simulink model "HopperPlant_Old"  (R2023b)
settings: Solver=VariableStepAuto  StartTime=0.0  StopTime=100  RelTol=1e-3
libraries: slpidlib x5, aerolibsim3d x2, shared6dof x1, sim3dlib x1
settings Model: Creator=xavie  LastModifiedBy=xavie

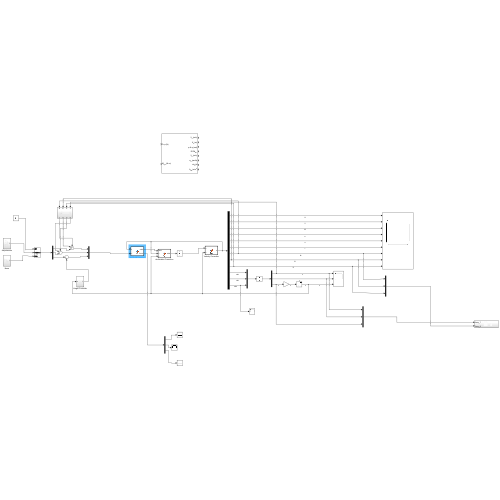
[thumbnail: Simulink's stored preview of the top-level diagram]
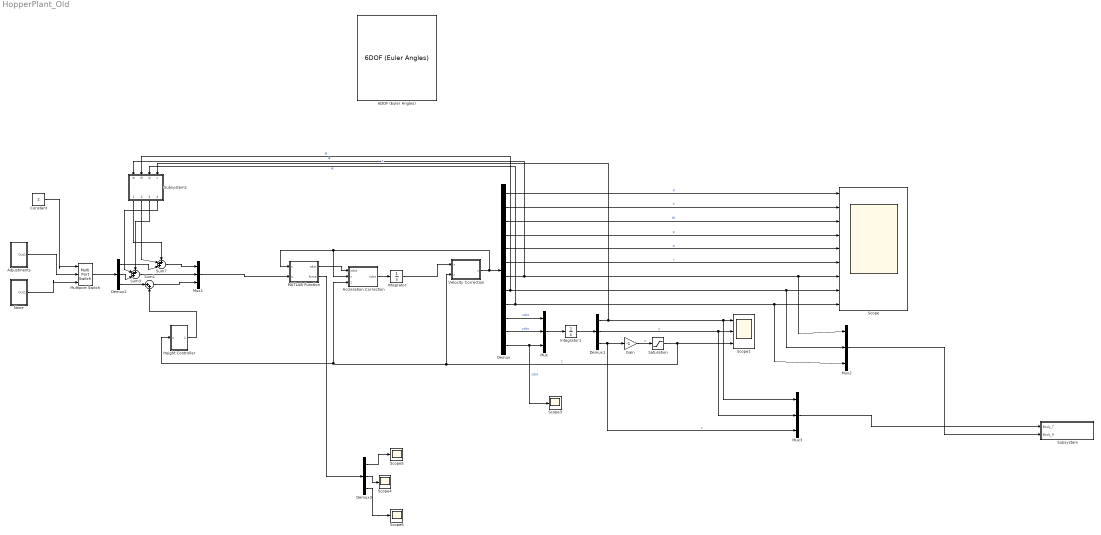
== system HopperPlant_Old ==
  6DOF (Euler Angles) : shared6dof/6DOF (Euler Angles)  units=Metric (MKS)  mtype=Fixed  rep=Euler Angles  xme_0=[0 0 0]  Vm_0=[0 0 0]  eul_0=[0 0 0]  pm_0=[0 0 0]  mass_0=1.0  mass_e=0.5  mass_f=2.0  inertia=eye(3)  inertia_e=eye(3)  inertia_f=2*eye(3)  k_quat=1.0  vre_flag=on  abi_flag=off  aMode=0  xme_statename=''  Vm_statename=''  eul_statename=''  quat_statename=''  pm_statename=''  mass_statename=''
  Accleration Correction : MATLAB Function  TreatAsAtomicUnit=on
  Adjustments : Subsystem
  Constant : Constant  Value=2
  Demux : Demux  Outputs=12
  Demux1 : Demux  Outputs=3
  Demux2 : Demux  Outputs=3
  Demux3 : Demux  Outputs=3
  Gain : Gain  Gain=-1
  Height Controller : Subsystem
  Integrator : Integrator  InitialCondition=[0;0;0;0;0;0;0;0;0;0;0;0]
  Integrator1 : Integrator  InitialCondition=[0;0;0]
  MATLAB Function : MATLAB Function  TreatAsAtomicUnit=on
  Multiport Switch : MultiPortSwitch  Inputs=2  SaturateOnIntegerOverflow=off  InputSameDT=off
  Mux{,1..3} (4 alike) : Mux  Inputs=3
  None : Subsystem
  Saturation : Saturate  UpperLimit=10000000000000000000000000000000000000000000  LowerLimit=0
  Scope : Scope  NumInputPorts=9
  Scope1 : Scope  NumInputPorts=3
  Scope{3..6} (4 alike) : Scope
  Subsystem : Subsystem
  Subsystem1 : Subsystem
  Sum1 : Sum  Inputs=|++
  Sum3 : Sum  Inputs=+++|
  Sum7 : Sum  Inputs=+++|
  Velocity Correction : MATLAB Function  TreatAsAtomicUnit=on
  wires:
  MATLAB Function/1(xdot) -> Accleration Correction/1("xdot ")
  Integrator/1 -> Velocity Correction/1("x ")
  Demux/1 -> Scope/1  "U"
  Demux/2 -> Scope/2  "V"
  Demux/3 -> Scope/3  "W"
  Demux/4 -> Scope/4  "p"
  Demux/5 -> Scope/5  "q"
  Demux/6 -> Scope/6  "r"
  Demux/7 -> Mux2/1, Scope/7, Subsystem1/1(Φ)  "Φ"
  Demux/8 -> Mux2/2, Scope/8, Subsystem1/2(Θ)  "Θ"
  Demux/9 -> Mux2/3, Scope/9, Subsystem1/3(Ψ)  "Ψ"
  Demux/10 -> Mux/1  "xdot"
  Demux/11 -> Mux/2  "ydot"
  Demux/12 -> Scope3/1, Mux/3  "zdot"
  Mux/1 -> Integrator1/1
  Integrator1/1 -> Demux1/1
  Demux1/1 -> Mux3/1, Scope1/1, Subsystem1/4(x)  "x"
  Demux1/2 -> Mux3/2, Scope1/2  "y"
  Demux1/3 -> Mux3/3, Gain/1  "z"
  Gain/1 -> Saturation/1  "z"
  Accleration Correction/1(xdot) -> Integrator/1
  Saturation/1 -> Velocity Correction/2(z), Height Controller/1(z), Accleration Correction/3(z), Scope1/3  "z"
  Velocity Correction/1(x) -> Accleration Correction/2(x), MATLAB Function/1(x), Demux/1
  Constant/1 -> Multiport Switch/1
  Adjustments/1(Out1) -> Multiport Switch/2
  None/1(Out1) -> Multiport Switch/3
  Multiport Switch/1 -> Demux2/1
  Demux2/3 -> Sum1/1
  Mux1/1 -> MATLAB Function/2(u)
  Sum1/1 -> Mux1/3
  MATLAB Function/2(force) -> Demux3/1
  Demux3/2 -> Scope4/1
  Demux3/1 -> Scope5/1
  Demux3/3 -> Scope6/1
  Mux2/1 -> Subsystem/2(Body_R)
  Mux3/1 -> Subsystem/1(Body_T)
  Sum3/1 -> Mux1/2
  Demux2/2 -> Sum3/3
  Demux2/1 -> Sum7/3
  Sum7/1 -> Mux1/1
  Height Controller/1(Out1) -> Sum1/2
  Subsystem1/1(Out1) -> Sum7/1
  Subsystem1/2(Out2) -> Sum7/2
  Subsystem1/3(Out3) -> Sum3/1
  Subsystem1/4(Out4) -> Sum3/2

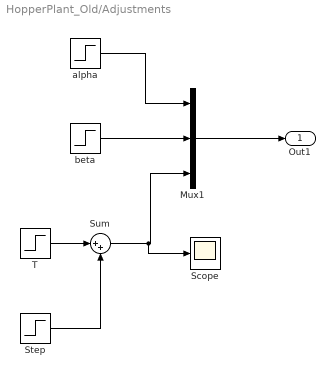
== system HopperPlant_Old/Adjustments ==
  Mux1 : Mux  Inputs=3
  Scope : Scope
  Step : Step  Time=10  After=-1500  SampleTime=0
  Sum : Sum  Inputs=|++
  T : Step  Time=0  After=1500  SampleTime=0
  alpha : Step  Time=0  After=pi/2  SampleTime=0
  beta : Step  Time=0  After=pi/2.001  SampleTime=0
  Out1 : Outport
  wires:
  alpha/1 -> Mux1/1
  Mux1/1 -> Out1/1
  beta/1 -> Mux1/2
  T/1 -> Sum/1
  Step/1 -> Sum/2
  Sum/1 -> Scope/1, Mux1/3

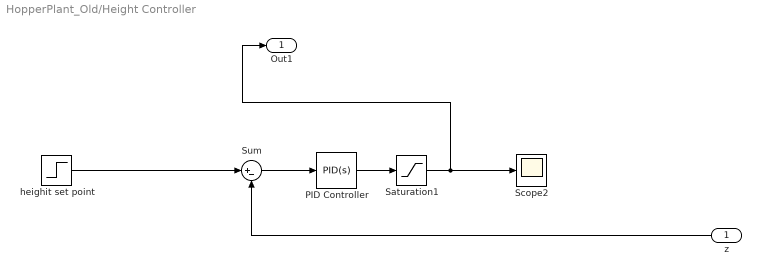
== system HopperPlant_Old/Height Controller ==
  z : Inport
  PID Controller : slpidlib/PID Controller  Controller=PID  Form=Parallel  TimeDomain=Continuous-time  UseExternalTs=off  SampleTime=-1  IntegratorMethod=Forward Euler  FilterMethod=Forward Euler  ControllerParametersSource=internal  P=40  I=2.1  UseKiTs=off  D=73  N=100  UseFilter=on  TunerSelectOption=Transfer Function Based (PID Tuner App)  InitialConditionSource=internal  InitialConditionForIntegrator=0  InitialConditionForFilter=0  DifferentiatorICPrevScaledInput=0  ExternalReset=none  TrackingMode=off  Kt=1  LimitOutput=off  SatLimitsSource=internal  UpperSaturationLimit=inf  LowerSaturationLimit=-inf  LinearizeAsGain=on  AntiWindupMode=none  Kb=1  LimitIntegrator=off  UpperIntegratorSaturationLimit=inf  LowerIntegratorSaturationLimit=-inf  POutMin=[]  POutMax=[]  IOutMin=[]  IOutMax=[]  DOutMin=[]  DOutMax=[]  NOutMin=[]  NOutMax=[]  SumOutMin=[]  SumOutMax=[]  SaturationOutMin=[]  SaturationOutMax=[]  PParamMin=[]  PParamMax=[]  IParamMin=[]  IParamMax=[]  DParamMin=[]  DParamMax=[]  NParamMin=[]  NParamMax=[]  KbParamMin=[]  KbParamMax=[]  KtParamMin=[]  KtParamMax=[]  KbOutMin=[]  KbOutMax=[]  KtOutMin=[]  KtOutMax=[]  IntegratorOutMin=[]  IntegratorOutMax=[]  FilterOutMin=[]  FilterOutMax=[]  SumI1OutMin=[]  SumI1OutMax=[]  SumI2OutMin=[]  SumI2OutMax=[]  SumI3OutMin=[]  SumI3OutMax=[]  SumI4OutMin=[]  SumI4OutMax=[]  SumDOutMin=[]  SumDOutMax=[]  DifferentiatorOutMin=[]  DifferentiatorOutMax=[]  FilterDiffOutCoefMin=[]  FilterDiffOutCoefMax=[]  ReciprocalOutMin=[]  ReciprocalOutMax=[]  SumDenOutMin=[]  SumDenOutMax=[]  SumNumOutMin=[]  SumNumOutMax=[]  DivideOutMin=[]  DivideOutMax=[]  UdiffTsProdOutMin=[]  UdiffTsProdOutMax=[]  NTsProdOutMin=[]  NTsProdOutMax=[]  UintegralTsProdOutMin=[]  UintegralTsProdOutMax=[]  UngainTsProdOutMin=[]  UngainTsProdOutMax=[]  ClampingZeroOutDataTypeStr=Inherit: Inherit via back propagation  ClampingZeroOutMin=[]  ClampingZeroOutMax=[]  FilterDenConstantOutDataTypeStr=Inherit: Inherit via back propagation  FilterDenConstantOutMin=[]  FilterDenConstantOutMax=[]  PCopyOutDataTypeStr=Inherit: Inherit via back propagation  PCopyOutMin=[]  PCopyOutMax=[]  NCopyOutDataTypeStr=Inherit: Inherit via back propagation  NCopyOutMin=[]  NCopyOutMax=[]  IntegratorContinuousStateAttributes=''  IntegratorStateMustResolveToSignalObject=off  IntegratorRTWStateStorageClass=Auto  FilterContinuousStateAttributes=''  FilterStateMustResolveToSignalObject=off  FilterRTWStateStorageClass=Auto  ParallelPVariant=InternalParameters  IdealPVariant=Disabled  IVariant=InternalParameters  DVariant=InternalParameters  IntegratorVariant=Continuous  SatVariant=Disabled  AWVariant=Passthrough  PCopyVariant=Disabled  TRVariant=Disabled  FdbkBlocksVariant=Forward  IdealPFdbkVariant=Disabled  SatFdbkVariant=Disabled  DerivativeFilterVariant=ContFilter  NVariant=InternalParameters  NCopyVariant=Disabled  FilterICVariant=InternalICsFilter  IntegratorICVariant=InternalICs  ExternalResetVariant=Disabled  TRSumVariant=Passthrough  SumFdbkVariant=Disabled  SumVariant=Sum_PID  TsampFilterVariant=InternalTs  TsampNgainVariant=Passthrough  TsampIntegralVariant=Disabled_SignalSpec  ExternalSaturationOutDataTypeStr=Inherit: Same as second input
  Saturation1 : Saturate  UpperLimit=1500  LowerLimit=0
  Scope2 : Scope
  Sum : Sum  Inputs=|+-
  heighit set point : Step  After=100  SampleTime=0
  Out1 : Outport
  wires:
  Saturation1/1 -> Out1/1, Scope2/1
  PID Controller/1 -> Saturation1/1
  Sum/1 -> PID Controller/1
  heighit set point/1 -> Sum/1
  z/1 -> Sum/2

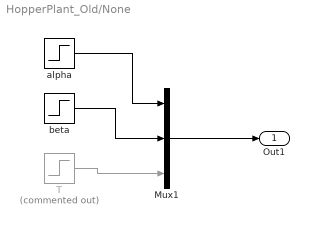
== system HopperPlant_Old/None ==
  Mux1 : Mux  Inputs=3
  T : Step  Commented=on  After=0  SampleTime=0
  alpha : Step  Time=0  After=0  SampleTime=0
  beta : Step  Time=0  After=pi/2.001  SampleTime=0
  Out1 : Outport
  wires:
  beta/1 -> Mux1/2
  T/1 -> Mux1/3
  alpha/1 -> Mux1/1
  Mux1/1 -> Out1/1

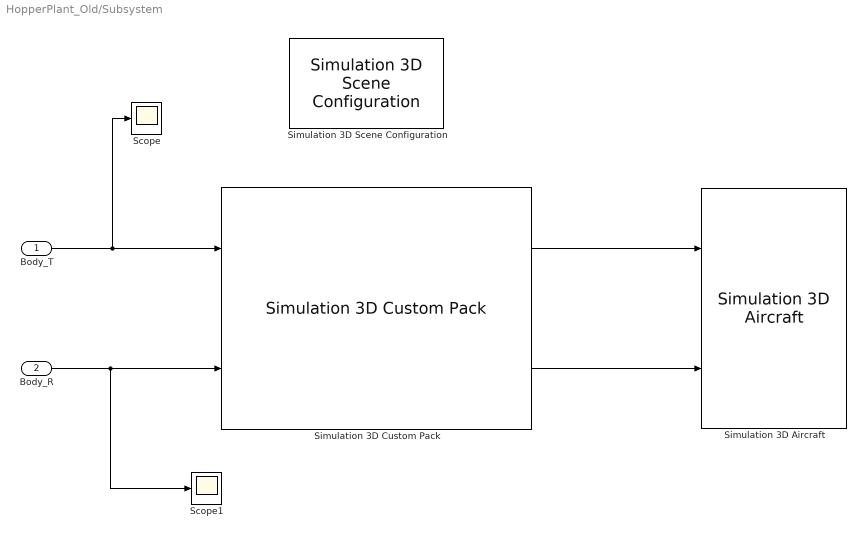
== system HopperPlant_Old/Subsystem ==
  Body_T : Inport
  Body_R : Inport  Port=2
  Scope : Scope
  Scope1 : Scope
  Simulation 3D Aircraft : aerolibsim3d/Simulation 3D Aircraft  Priority=-1  Mesh=Custom  MeshPath=/MathWorksAerospaceContent/Vehicles/Aircraft/Custom/Mesh/SK_HL20.SK_HL20  MeshPathAT=/MathWorksAerospaceContent/Vehicles/Aircraft/AirTransport/Mesh/SK_AirTransport.SK_AirTransport  MeshPathGA=/MathWorksAerospaceContent/Vehicles/Aircraft/GeneralAviation/Mesh/SK_GeneralAviation.SK_GeneralAviation  AircraftColor=White  ActorName=SimulinkVehicle2  Translation=[0, 300, 0; zeros( 56, 3 )]  Rotation=zeros( 57, 3 )  IsGHSensorEnabled=off  AreGHRaysVisible=off  IsOutputReshapeEnabled=off  GHRayLength=5000  GHBodyOffset=0.90  GHFrontTireRadius=0.21  GHLeftTireRadius=0.21  GHRightTireRadius=0.21  WoWSensorTolerance=0.05  LightsConfig=Automatic lights  LandingLightIntensity=300000  LandingLightConeAngle=15  CustomLeftLandingLightLocation=[0 0 0]  CustomLeftLandingLightOrientation=[0 0 0]  CustomRightLandingLightLocation=[0 0 0]  CustomRightLandingLightOrientation=[0 0 0]  TaxiLightIntensity=150000  TaxiLightConeAngle=36  CustomTaxiLightLocation=[0 0 0]  CustomTaxiLightOrientation=[0 0 0]  NavLightIntensity=500  PositionLightIntensity=500  StrobeLightIntensity=5000  WingtipStrobePeriod=1.5  WingtipStrobePulseWidth=6  TailStrobePeriod=1.5  TailStrobePulseWidth=6  BeaconLightIntensity=4000  BeaconPeriod=1.5  BeaconPulseWidth=10  SampleTime=-1  ActorType=SimulinkVehicle  ID=2  aMode=0  ActorTag=SimulinkVehicle2
  Simulation 3D Custom Pack : aerolibsim3d/Simulation 3D Custom Pack  Engine1_T=off  Engine1_R=off  Engine1_Prop_T=off  Engine1_Prop_R=off  Engine2_T=off  Engine2_R=off  Engine2_Prop_T=off  Engine2_Prop_R=off  Engine3_T=off  Engine3_R=off  Engine3_Prop_T=off  Engine3_Prop_R=off  Engine4_T=off  Engine4_R=off  Engine4_Prop_T=off  Engine4_Prop_R=off  Engine5_T=off  Engine5_R=off  Engine5_Prop_T=off  Engine5_Prop_R=off  Engine6_T=off  Engine6_R=off  Engine6_Prop_T=off  Engine6_Prop_R=off  Engine7_T=off  Engine7_R=off  Engine7_Prop_T=off  Engine7_Prop_R=off  Engine8_T=off  Engine8_R=off  Engine8_Prop_T=off  Engine8_Prop_R=off  Engine9_T=off  Engine9_R=off  Engine9_Prop_T=off  Engine9_Prop_R=off  Engine10_T=off  Engine10_R=off  Engine10_Prop_T=off  Engine10_Prop_R=off  Engine11_T=off  Engine11_R=off  Engine11_Prop_T=off  Engine11_Prop_R=off  Engine12_T=off  Engine12_R=off  Engine12_Prop_T=off  Engine12_Prop_R=off  Engine13_T=off  Engine13_R=off  Engine13_Prop_T=off  Engine13_Prop_R=off  Engine14_T=off  Engine14_R=off  Engine14_Prop_T=off  Engine14_Prop_R=off  Engine15_T=off  Engine15_R=off  Engine15_Prop_T=off  Engine15_Prop_R=off  Engine16_T=off  Engine16_R=off  Engine16_Prop_T=off  Engine16_Prop_R=off  Wing1_T=off  Wing1_R=off  Wing1_Left_Flap_T=off  Wing1_Left_Flap_R=off  Wing1_Right_Flap_T=off  Wing1_Right_Flap_R=off  Wing1_Left_Aileron_T=off  Wing1_Left_Aileron_R=off  Wing1_Right_Aileron_T=off  Wing1_Right_Aileron_R=off  Wing1_Left_Spoiler_T=off  Wing1_Left_Spoiler_R=off  Wing1_Right_Spoiler_T=off  Wing1_Right_Spoiler_R=off  Wing2_T=off  Wing2_R=off  Wing2_Left_Flap_T=off  Wing2_Left_Flap_R=off  Wing2_Right_Flap_T=off  Wing2_Right_Flap_R=off  Horizontal_Stab_T=off  Horizontal_Stab_R=off  Left_Elevator_T=off  Left_Elevator_R=off  Right_Elevator_T=off  Right_Elevator_R=off  Left_Rudder_T=off  Left_Rudder_R=off  Right_Rudder_T=off  Right_Rudder_R=off  Nose_Gear_T=off  Nose_Gear_R=off  Nose_Wheel_T=off  Nose_Wheel_R=off  Nose_Gear_Door_T=off  Nose_Gear_Door_R=off  Left_Gear_T=off  Left_Gear_R=off  Left_Wheel_T=off  Left_Wheel_R=off  Left_Gear_Door_T=off  Left_Gear_Door_R=off  Right_Gear_T=off  Right_Gear_R=off  Right_Wheel_T=off  Right_Wheel_R=off  Right_Gear_Door_T=off  Right_Gear_Door_R=off  AdjustForCesium=off  Heading0=90
  Simulation 3D Scene Configuration : sim3dlib/Simulation 3D Scene Configuration  Priority=0  ProjectFormat=Default Scenes  SceneDesc=Airport  ProjectName=E:\Matlab 2023b\toolbox\shared\sim3d_projects\automotive_project_windows\UE\WindowsNoEditor\VehicleSimulation.exe  ScenePath=/Game/Maps/HwStrght  EnableOpenDRIVE=off  vehTagList={'Custom';'Scene Origin';'SimulinkVehicle2'}  vehTag=SimulinkVehicle2  FreeCameraInitialTranslation=[0, 0, 0]  FreeCameraDefaultInitialTranslation=[-6, 0, 2]  FreeCameraInitialRotation=[0, 0, 0]  FreeCameraDefaultInitialRotation=[0, -15, 0]  OpVisEn=off  Ts=1/60  EnableWindow=on  EnableRemoteAccess=off  EnableWeather=off  SunAltitude=40.0  SunAzimuth=90  clouds=10  wind=1  fog=0  rain=0  EnableGeospatial=off  OriginHeight=200  OriginLatitude=40.744652  OriginLongitude=-73.988864  MapStyle=Aerial  AdditionalAssetIDs=[]  UseAdvancedSunSky=off  SolarTime=11  TimeZone=-5  Day=21  Month=9  Year=2022  UseDaylightSavingTime=on  DSTStartDay=10  DSTStartMonth=3  DSTEndDay=3  DSTEndMonth=11  DSTSwitchHour=2  sensorTag=MainCamera1  sensorId=1  sensorName=MainCamera1  mountLoc=Origin  offsetFlag=off  tmountOffset=[0, 0, 0]  rmountOffset=[0, 0, 0]  HorizontalResolution=1280  VerticalResolution=720  HorizontalFOV=60  mountPoint=[0 0 0]  mountOrientation=[0 0 0]  aMode=0  ID=1  GeoTrigger=Inactive
      settings: LibrarySourceBlock=aerolibsim3d/Simulation 3D Scene Configuration
  wires:
  Body_R/1 -> Scope1/1, Simulation 3D Custom Pack/2
  Simulation 3D Custom Pack/2 -> Simulation 3D Aircraft/2
  Body_T/1 -> Scope/1, Simulation 3D Custom Pack/1
  Simulation 3D Custom Pack/1 -> Simulation 3D Aircraft/1

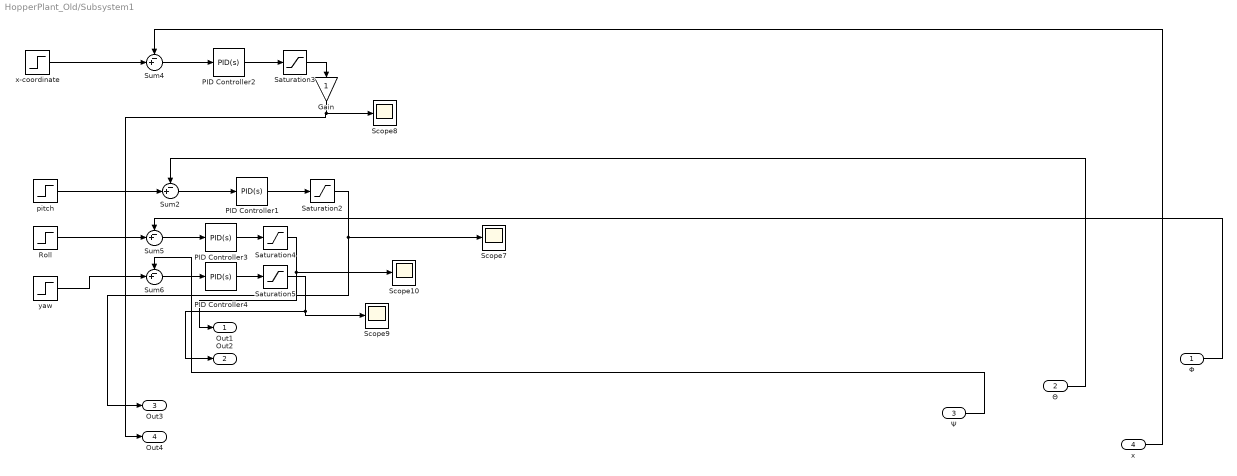
== system HopperPlant_Old/Subsystem1 ==
  Φ : Inport
  Θ : Inport  Port=2
  Ψ : Inport  Port=3
  x : Inport  Port=4
  Gain : Gain
  PID Controller1 : slpidlib/PID Controller  Controller=PID  Form=Parallel  TimeDomain=Continuous-time  UseExternalTs=off  SampleTime=-1  IntegratorMethod=Forward Euler  FilterMethod=Forward Euler  ControllerParametersSource=internal  P=-0.01  I=-0.001  UseKiTs=off  D=-0.15  N=100  UseFilter=on  TunerSelectOption=Transfer Function Based (PID Tuner App)  InitialConditionSource=internal  InitialConditionForIntegrator=0  InitialConditionForFilter=0  DifferentiatorICPrevScaledInput=0  ExternalReset=none  TrackingMode=off  Kt=1  LimitOutput=off  SatLimitsSource=internal  UpperSaturationLimit=inf  LowerSaturationLimit=-inf  LinearizeAsGain=on  AntiWindupMode=none  Kb=1  LimitIntegrator=off  UpperIntegratorSaturationLimit=inf  LowerIntegratorSaturationLimit=-inf  POutMin=[]  POutMax=[]  IOutMin=[]  IOutMax=[]  DOutMin=[]  DOutMax=[]  NOutMin=[]  NOutMax=[]  SumOutMin=[]  SumOutMax=[]  SaturationOutMin=[]  SaturationOutMax=[]  PParamMin=[]  PParamMax=[]  IParamMin=[]  IParamMax=[]  DParamMin=[]  DParamMax=[]  NParamMin=[]  NParamMax=[]  KbParamMin=[]  KbParamMax=[]  KtParamMin=[]  KtParamMax=[]  KbOutMin=[]  KbOutMax=[]  KtOutMin=[]  KtOutMax=[]  IntegratorOutMin=[]  IntegratorOutMax=[]  FilterOutMin=[]  FilterOutMax=[]  SumI1OutMin=[]  SumI1OutMax=[]  SumI2OutMin=[]  SumI2OutMax=[]  SumI3OutMin=[]  SumI3OutMax=[]  SumI4OutMin=[]  SumI4OutMax=[]  SumDOutMin=[]  SumDOutMax=[]  DifferentiatorOutMin=[]  DifferentiatorOutMax=[]  FilterDiffOutCoefMin=[]  FilterDiffOutCoefMax=[]  ReciprocalOutMin=[]  ReciprocalOutMax=[]  SumDenOutMin=[]  SumDenOutMax=[]  SumNumOutMin=[]  SumNumOutMax=[]  DivideOutMin=[]  DivideOutMax=[]  UdiffTsProdOutMin=[]  UdiffTsProdOutMax=[]  NTsProdOutMin=[]  NTsProdOutMax=[]  UintegralTsProdOutMin=[]  UintegralTsProdOutMax=[]  UngainTsProdOutMin=[]  UngainTsProdOutMax=[]  ClampingZeroOutDataTypeStr=Inherit: Inherit via back propagation  ClampingZeroOutMin=[]  ClampingZeroOutMax=[]  FilterDenConstantOutDataTypeStr=Inherit: Inherit via back propagation  FilterDenConstantOutMin=[]  FilterDenConstantOutMax=[]  PCopyOutDataTypeStr=Inherit: Inherit via back propagation  PCopyOutMin=[]  PCopyOutMax=[]  NCopyOutDataTypeStr=Inherit: Inherit via back propagation  NCopyOutMin=[]  NCopyOutMax=[]  IntegratorContinuousStateAttributes=''  IntegratorStateMustResolveToSignalObject=off  IntegratorRTWStateStorageClass=Auto  FilterContinuousStateAttributes=''  FilterStateMustResolveToSignalObject=off  FilterRTWStateStorageClass=Auto  ParallelPVariant=InternalParameters  IdealPVariant=Disabled  IVariant=InternalParameters  DVariant=InternalParameters  IntegratorVariant=Continuous  SatVariant=Disabled  AWVariant=Passthrough  PCopyVariant=Disabled  TRVariant=Disabled  FdbkBlocksVariant=Forward  IdealPFdbkVariant=Disabled  SatFdbkVariant=Disabled  DerivativeFilterVariant=ContFilter  NVariant=InternalParameters  NCopyVariant=Disabled  FilterICVariant=InternalICsFilter  IntegratorICVariant=InternalICs  ExternalResetVariant=Disabled  TRSumVariant=Passthrough  SumFdbkVariant=Disabled  SumVariant=Sum_PID  TsampFilterVariant=InternalTs  TsampNgainVariant=Passthrough  TsampIntegralVariant=Disabled_SignalSpec  ExternalSaturationOutDataTypeStr=Inherit: Same as second input
  PID Controller2 : slpidlib/PID Controller  Controller=PID  Form=Parallel  TimeDomain=Continuous-time  UseExternalTs=off  SampleTime=-1  IntegratorMethod=Forward Euler  FilterMethod=Forward Euler  ControllerParametersSource=internal  P=-0.000075  I=-0.000033  UseKiTs=off  D=-0.021  N=100  UseFilter=on  TunerSelectOption=Transfer Function Based (PID Tuner App)  InitialConditionSource=internal  InitialConditionForIntegrator=0  InitialConditionForFilter=0  DifferentiatorICPrevScaledInput=0  ExternalReset=none  TrackingMode=off  Kt=1  LimitOutput=off  SatLimitsSource=internal  UpperSaturationLimit=inf  LowerSaturationLimit=-inf  LinearizeAsGain=on  AntiWindupMode=none  Kb=1  LimitIntegrator=off  UpperIntegratorSaturationLimit=inf  LowerIntegratorSaturationLimit=-inf  POutMin=[]  POutMax=[]  IOutMin=[]  IOutMax=[]  DOutMin=[]  DOutMax=[]  NOutMin=[]  NOutMax=[]  SumOutMin=[]  SumOutMax=[]  SaturationOutMin=[]  SaturationOutMax=[]  PParamMin=[]  PParamMax=[]  IParamMin=[]  IParamMax=[]  DParamMin=[]  DParamMax=[]  NParamMin=[]  NParamMax=[]  KbParamMin=[]  KbParamMax=[]  KtParamMin=[]  KtParamMax=[]  KbOutMin=[]  KbOutMax=[]  KtOutMin=[]  KtOutMax=[]  IntegratorOutMin=[]  IntegratorOutMax=[]  FilterOutMin=[]  FilterOutMax=[]  SumI1OutMin=[]  SumI1OutMax=[]  SumI2OutMin=[]  SumI2OutMax=[]  SumI3OutMin=[]  SumI3OutMax=[]  SumI4OutMin=[]  SumI4OutMax=[]  SumDOutMin=[]  SumDOutMax=[]  DifferentiatorOutMin=[]  DifferentiatorOutMax=[]  FilterDiffOutCoefMin=[]  FilterDiffOutCoefMax=[]  ReciprocalOutMin=[]  ReciprocalOutMax=[]  SumDenOutMin=[]  SumDenOutMax=[]  SumNumOutMin=[]  SumNumOutMax=[]  DivideOutMin=[]  DivideOutMax=[]  UdiffTsProdOutMin=[]  UdiffTsProdOutMax=[]  NTsProdOutMin=[]  NTsProdOutMax=[]  UintegralTsProdOutMin=[]  UintegralTsProdOutMax=[]  UngainTsProdOutMin=[]  UngainTsProdOutMax=[]  ClampingZeroOutDataTypeStr=Inherit: Inherit via back propagation  ClampingZeroOutMin=[]  ClampingZeroOutMax=[]  FilterDenConstantOutDataTypeStr=Inherit: Inherit via back propagation  FilterDenConstantOutMin=[]  FilterDenConstantOutMax=[]  PCopyOutDataTypeStr=Inherit: Inherit via back propagation  PCopyOutMin=[]  PCopyOutMax=[]  NCopyOutDataTypeStr=Inherit: Inherit via back propagation  NCopyOutMin=[]  NCopyOutMax=[]  IntegratorContinuousStateAttributes=''  IntegratorStateMustResolveToSignalObject=off  IntegratorRTWStateStorageClass=Auto  FilterContinuousStateAttributes=''  FilterStateMustResolveToSignalObject=off  FilterRTWStateStorageClass=Auto  ParallelPVariant=InternalParameters  IdealPVariant=Disabled  IVariant=InternalParameters  DVariant=InternalParameters  IntegratorVariant=Continuous  SatVariant=Disabled  AWVariant=Passthrough  PCopyVariant=Disabled  TRVariant=Disabled  FdbkBlocksVariant=Forward  IdealPFdbkVariant=Disabled  SatFdbkVariant=Disabled  DerivativeFilterVariant=ContFilter  NVariant=InternalParameters  NCopyVariant=Disabled  FilterICVariant=InternalICsFilter  IntegratorICVariant=InternalICs  ExternalResetVariant=Disabled  TRSumVariant=Passthrough  SumFdbkVariant=Disabled  SumVariant=Sum_PID  TsampFilterVariant=InternalTs  TsampNgainVariant=Passthrough  TsampIntegralVariant=Disabled_SignalSpec  ExternalSaturationOutDataTypeStr=Inherit: Same as second input
  PID Controller3 : slpidlib/PID Controller  Controller=PID  Form=Parallel  TimeDomain=Continuous-time  UseExternalTs=off  SampleTime=-1  IntegratorMethod=Forward Euler  FilterMethod=Forward Euler  ControllerParametersSource=internal  P=0  I=0  UseKiTs=off  D=0  N=100  UseFilter=on  TunerSelectOption=Transfer Function Based (PID Tuner App)  InitialConditionSource=internal  InitialConditionForIntegrator=0  InitialConditionForFilter=0  DifferentiatorICPrevScaledInput=0  ExternalReset=none  TrackingMode=off  Kt=1  LimitOutput=off  SatLimitsSource=internal  UpperSaturationLimit=inf  LowerSaturationLimit=-inf  LinearizeAsGain=on  AntiWindupMode=none  Kb=1  LimitIntegrator=off  UpperIntegratorSaturationLimit=inf  LowerIntegratorSaturationLimit=-inf  POutMin=[]  POutMax=[]  IOutMin=[]  IOutMax=[]  DOutMin=[]  DOutMax=[]  NOutMin=[]  NOutMax=[]  SumOutMin=[]  SumOutMax=[]  SaturationOutMin=[]  SaturationOutMax=[]  PParamMin=[]  PParamMax=[]  IParamMin=[]  IParamMax=[]  DParamMin=[]  DParamMax=[]  NParamMin=[]  NParamMax=[]  KbParamMin=[]  KbParamMax=[]  KtParamMin=[]  KtParamMax=[]  KbOutMin=[]  KbOutMax=[]  KtOutMin=[]  KtOutMax=[]  IntegratorOutMin=[]  IntegratorOutMax=[]  FilterOutMin=[]  FilterOutMax=[]  SumI1OutMin=[]  SumI1OutMax=[]  SumI2OutMin=[]  SumI2OutMax=[]  SumI3OutMin=[]  SumI3OutMax=[]  SumI4OutMin=[]  SumI4OutMax=[]  SumDOutMin=[]  SumDOutMax=[]  DifferentiatorOutMin=[]  DifferentiatorOutMax=[]  FilterDiffOutCoefMin=[]  FilterDiffOutCoefMax=[]  ReciprocalOutMin=[]  ReciprocalOutMax=[]  SumDenOutMin=[]  SumDenOutMax=[]  SumNumOutMin=[]  SumNumOutMax=[]  DivideOutMin=[]  DivideOutMax=[]  UdiffTsProdOutMin=[]  UdiffTsProdOutMax=[]  NTsProdOutMin=[]  NTsProdOutMax=[]  UintegralTsProdOutMin=[]  UintegralTsProdOutMax=[]  UngainTsProdOutMin=[]  UngainTsProdOutMax=[]  ClampingZeroOutDataTypeStr=Inherit: Inherit via back propagation  ClampingZeroOutMin=[]  ClampingZeroOutMax=[]  FilterDenConstantOutDataTypeStr=Inherit: Inherit via back propagation  FilterDenConstantOutMin=[]  FilterDenConstantOutMax=[]  PCopyOutDataTypeStr=Inherit: Inherit via back propagation  PCopyOutMin=[]  PCopyOutMax=[]  NCopyOutDataTypeStr=Inherit: Inherit via back propagation  NCopyOutMin=[]  NCopyOutMax=[]  IntegratorContinuousStateAttributes=''  IntegratorStateMustResolveToSignalObject=off  IntegratorRTWStateStorageClass=Auto  FilterContinuousStateAttributes=''  FilterStateMustResolveToSignalObject=off  FilterRTWStateStorageClass=Auto  ParallelPVariant=InternalParameters  IdealPVariant=Disabled  IVariant=InternalParameters  DVariant=InternalParameters  IntegratorVariant=Continuous  SatVariant=Disabled  AWVariant=Passthrough  PCopyVariant=Disabled  TRVariant=Disabled  FdbkBlocksVariant=Forward  IdealPFdbkVariant=Disabled  SatFdbkVariant=Disabled  DerivativeFilterVariant=ContFilter  NVariant=InternalParameters  NCopyVariant=Disabled  FilterICVariant=InternalICsFilter  IntegratorICVariant=InternalICs  ExternalResetVariant=Disabled  TRSumVariant=Passthrough  SumFdbkVariant=Disabled  SumVariant=Sum_PID  TsampFilterVariant=InternalTs  TsampNgainVariant=Passthrough  TsampIntegralVariant=Disabled_SignalSpec  ExternalSaturationOutDataTypeStr=Inherit: Same as second input
  PID Controller4 : slpidlib/PID Controller  Controller=PID  Form=Parallel  TimeDomain=Continuous-time  UseExternalTs=off  SampleTime=-1  IntegratorMethod=Forward Euler  FilterMethod=Forward Euler  ControllerParametersSource=internal  P=0  I=0  UseKiTs=off  D=0  N=100  UseFilter=on  TunerSelectOption=Transfer Function Based (PID Tuner App)  InitialConditionSource=internal  InitialConditionForIntegrator=0  InitialConditionForFilter=0  DifferentiatorICPrevScaledInput=0  ExternalReset=none  TrackingMode=off  Kt=1  LimitOutput=off  SatLimitsSource=internal  UpperSaturationLimit=inf  LowerSaturationLimit=-inf  LinearizeAsGain=on  AntiWindupMode=none  Kb=1  LimitIntegrator=off  UpperIntegratorSaturationLimit=inf  LowerIntegratorSaturationLimit=-inf  POutMin=[]  POutMax=[]  IOutMin=[]  IOutMax=[]  DOutMin=[]  DOutMax=[]  NOutMin=[]  NOutMax=[]  SumOutMin=[]  SumOutMax=[]  SaturationOutMin=[]  SaturationOutMax=[]  PParamMin=[]  PParamMax=[]  IParamMin=[]  IParamMax=[]  DParamMin=[]  DParamMax=[]  NParamMin=[]  NParamMax=[]  KbParamMin=[]  KbParamMax=[]  KtParamMin=[]  KtParamMax=[]  KbOutMin=[]  KbOutMax=[]  KtOutMin=[]  KtOutMax=[]  IntegratorOutMin=[]  IntegratorOutMax=[]  FilterOutMin=[]  FilterOutMax=[]  SumI1OutMin=[]  SumI1OutMax=[]  SumI2OutMin=[]  SumI2OutMax=[]  SumI3OutMin=[]  SumI3OutMax=[]  SumI4OutMin=[]  SumI4OutMax=[]  SumDOutMin=[]  SumDOutMax=[]  DifferentiatorOutMin=[]  DifferentiatorOutMax=[]  FilterDiffOutCoefMin=[]  FilterDiffOutCoefMax=[]  ReciprocalOutMin=[]  ReciprocalOutMax=[]  SumDenOutMin=[]  SumDenOutMax=[]  SumNumOutMin=[]  SumNumOutMax=[]  DivideOutMin=[]  DivideOutMax=[]  UdiffTsProdOutMin=[]  UdiffTsProdOutMax=[]  NTsProdOutMin=[]  NTsProdOutMax=[]  UintegralTsProdOutMin=[]  UintegralTsProdOutMax=[]  UngainTsProdOutMin=[]  UngainTsProdOutMax=[]  ClampingZeroOutDataTypeStr=Inherit: Inherit via back propagation  ClampingZeroOutMin=[]  ClampingZeroOutMax=[]  FilterDenConstantOutDataTypeStr=Inherit: Inherit via back propagation  FilterDenConstantOutMin=[]  FilterDenConstantOutMax=[]  PCopyOutDataTypeStr=Inherit: Inherit via back propagation  PCopyOutMin=[]  PCopyOutMax=[]  NCopyOutDataTypeStr=Inherit: Inherit via back propagation  NCopyOutMin=[]  NCopyOutMax=[]  IntegratorContinuousStateAttributes=''  IntegratorStateMustResolveToSignalObject=off  IntegratorRTWStateStorageClass=Auto  FilterContinuousStateAttributes=''  FilterStateMustResolveToSignalObject=off  FilterRTWStateStorageClass=Auto  ParallelPVariant=InternalParameters  IdealPVariant=Disabled  IVariant=InternalParameters  DVariant=InternalParameters  IntegratorVariant=Continuous  SatVariant=Disabled  AWVariant=Passthrough  PCopyVariant=Disabled  TRVariant=Disabled  FdbkBlocksVariant=Forward  IdealPFdbkVariant=Disabled  SatFdbkVariant=Disabled  DerivativeFilterVariant=ContFilter  NVariant=InternalParameters  NCopyVariant=Disabled  FilterICVariant=InternalICsFilter  IntegratorICVariant=InternalICs  ExternalResetVariant=Disabled  TRSumVariant=Passthrough  SumFdbkVariant=Disabled  SumVariant=Sum_PID  TsampFilterVariant=InternalTs  TsampNgainVariant=Passthrough  TsampIntegralVariant=Disabled_SignalSpec  ExternalSaturationOutDataTypeStr=Inherit: Same as second input
  Roll : Step  SampleTime=0
  Saturation2 : Saturate  UpperLimit=pi/2  LowerLimit=-pi/2
  Saturation3 : Saturate  UpperLimit=pi/2  LowerLimit=-pi/2
  Saturation4 : Saturate  UpperLimit=pi  LowerLimit=-pi
  Saturation5 : Saturate  UpperLimit=pi  LowerLimit=-pi
  Scope{7..10} (4 alike) : Scope
  Sum{2,4..6} (4 alike) : Sum  Inputs=-+|
  pitch : Step  Time=0  After=0  SampleTime=0
  x-coordinate : Step  Time=0  After=0  SampleTime=0
  yaw : Step  SampleTime=0
  Out1 : Outport
  Out2 : Outport  Port=2
  Out3 : Outport  Port=3
  Out4 : Outport  Port=4
  wires:
  Sum2/1 -> PID Controller1/1
  Saturation3/1 -> Gain/1
  Sum5/1 -> PID Controller3/1
  pitch/1 -> Sum2/2
  Ψ/1 -> Sum6/1
  Roll/1 -> Sum5/2
  yaw/1 -> Sum6/2
  Sum4/1 -> PID Controller2/1
  PID Controller1/1 -> Saturation2/1
  Saturation2/1 -> Out3/1, Scope7/1
  PID Controller4/1 -> Saturation5/1
  Sum6/1 -> PID Controller4/1
  PID Controller3/1 -> Saturation4/1
  PID Controller2/1 -> Saturation3/1
  x-coordinate/1 -> Sum4/2
  Saturation5/1 -> Out2/1, Scope9/1
  Θ/1 -> Sum2/1
  Saturation4/1 -> Out1/1, Scope10/1
  Φ/1 -> Sum5/1
  x/1 -> Sum4/1
  Gain/1 -> Out4/1, Scope8/1

== matlab function HopperPlant_Old/Accleration Correction ==
  data: xdot input; x input; xdot output; z input
function xdot = fcn(xdot,x, z)

phi=x(7);
theta=x(8);
psi=x(9);
T_etob=[cos(theta)*cos(psi),cos(theta)*sin(psi),-sin(theta);
    sin(theta)*sin(phi)*cos(phi)-sin(psi)*cos(phi),sin(psi)*sin(theta)*sin(phi)+cos(psi)*cos(phi), sin(phi)*cos(theta);
    sin(theta)*cos(phi)*cos(psi)+sin(psi)*sin(phi), sin(phi)*sin(theta)*cos(phi)-cos(psi)*sin(theta), cos(phi)*cos(theta)];
zddot=xdot(end);

if z <= 0 && zddot > 0
    xdot(end)=0;
    xdot(end-1)=0;
    xdot(end-2)=0;
    xdot(1:3)=T_etob*[xdot(end-2);xdot(end-1);xdot(end)];
    
end

== matlab function HopperPlant_Old/MATLAB Function ==
  data: x input; u input; xdot output; force output
function [xdot,force]  = fcn(x, u)
%{
Takes in thrust, angles of thrust, x and outputs xdot
Body axis is defined as z being the in the direction of gravity when pitch
is zero

m - mass-kg
I - moment of intertia - kg m^2
cg - centre of gravity - m
thrust position - m
U - body axis x velocity - m/s
V - body axis y velocity - m/s
W - body axis z velocity - m/s
p - body axis roll rate - rad/s
q - body axis pitch rate - rad/s
r - body axis yaw rate - rad/s
phi - earth axis roll - rad
theta - earth axis pitch - rad
psi - earth axis yaw - rad
alpha - thrust rotation angle 
%}


%%Control input
alpha=u(1); 
beta=u(2);
% T1=u(3);
% T2=u(4);
T=u(3);

 % alpha=0; 
 % beta=0;
 % T1=0;
 % T2=0;
 % T=T1+T2;

%%states
U=x(1);
V=x(2);
W=x(3);
p=x(4);
q=x(5);
r=x(6);
phi=x(7);
theta=x(8);
psi=x(9);


%%Constants
T_etob=[cos(theta)*cos(psi), sin(theta)*sin(phi)*cos(psi)-cos(phi)*sin(psi), cos(phi)*sin(theta)*cos(psi)+sin(phi)*sin(psi);
    cos(theta)*sin(psi), sin(phi)*sin(theta)*sin(psi)+cos(phi)*cos(psi), cos(phi)*sin(theta)*cos(psi)-sin(phi)*cos(psi);
    -sin(theta),sin(phi)*cos(theta), cos(phi)*cos(theta)];
gb=9.81;
ge=T_etob*[0;0;gb];
gx=ge(1);
gy=ge(2);
gz=ge(3);

%%Mass and inertia

m=100;
Ixx=units(2.671e10,'g*mm^2','kg*m^2');
Iyy=units(2.671e10,'g*mm^2','kg*m^2');
Izz=units(4.915e09,'g*mm^2','kg*m^2');
Ixz=units(-1.112e06,'g*mm^2','kg*m^2');

% Ixx=units(4.915e09,'g*mm^2','kg*m^2');
% Iyy=units(2.614e10,'g*mm^2','kg*m^2');
% Izz=units(1.614e10,'g*mm^2','kg*m^2');
% Ixz=units(-1.629e08,'g*mm^2','kg*m^2');

cg=[0,0,units(800,'mm','m')];
thrust_pos=[units(0,'mm','m'),units(0,'mm','m'),units(1350,'mm','m')];

%%Forces

 Tx=T*cos(beta)*cos(alpha);
 Ty=T*cos(beta)*sin(alpha);
 Tz=-T*sin(beta);

 Fx=Tx+m*gx;
 Fy=Ty+m*gy;
 Fz=Tz+m*gz;



%%Rotational moments
lx=thrust_pos(1)-cg(1);
ly=thrust_pos(2)-cg(2);
lz=thrust_pos(3)-cg(3);

L=ly*Tz-lz*Ty;
M=lx*Tz+lz*Tx;
N=-lx*Ty-ly*Tx;


%%Compute xdot
Udot=Fx/m-(W*q-V*r);
Vdot=Fy/m-(U*r-p*W);
Wdot=Fz/m-(V*p-U*q);

A=L+Ixz*q*p-(Izz-Iyy)*q*r;
B=M-Ixz*(p^2-r^2)-(Ixx-Izz)*p*r;
C=N-Ixz*q*r-(Iyy-Ixx)*p*q;


pr_dot=[Ixx, -Ixz; -Ixz, Izz]\[A;C];
pdot=pr_dot(1);
qdot=B/Iyy;
rdot=pr_dot(2);

% pdot=(L-q*r*(Izz-Iyy))/Ixx;
% qdot=(M-r*p*(Ixx-Izz))/Iyy;
% rdot=(N-p*q*(Iyy-Ixx))/Izz;

% Compute Euler angles
AngleCon_btoe=[1 sin(phi)*tan(theta), cos(phi)*tan(theta);
    0, cos(phi), -sin(phi); ...
    0, sin(phi)*sec(theta), cos(phi)*sec(theta)];


EulerAngledot=AngleCon_btoe*[p;q;r];
 T_btoe=transpose(T_etob);
Earthacceleration=T_etob\[Udot;Vdot;Wdot];
convertg=T_btoe*[Fx;Fy;Fz];

xdot=[Udot;Vdot;Wdot;pdot;qdot; rdot;EulerAngledot;Earthacceleration];
force=[Udot, Vdot, Wdot];

== matlab function HopperPlant_Old/Velocity Correction ==
  data: x input; x output; z input
function x = fcn(x, z)

phi=x(7);
theta=x(8);
psi=x(9);
T_etob=[cos(theta)*cos(psi),cos(theta)*sin(psi),-sin(theta);
    sin(theta)*sin(phi)*cos(phi)-sin(psi)*cos(phi),sin(psi)*sin(theta)*sin(phi)+cos(psi)*cos(phi), sin(phi)*cos(theta);
    sin(theta)*cos(phi)*cos(psi)+sin(psi)*sin(phi), sin(phi)*sin(theta)*cos(phi)-cos(psi)*sin(theta), cos(phi)*cos(theta)];
zdot=x(end);

if z <= 0 && zdot > 0
    x(end)=0;
    x(end-1)=0;
    x(end-2)=0;
    x(3)=0;
    x(4)=0;
    x(5)=0;
    x(1:3)=T_etob*[x(end-2);x(end-1);x(end)];
   
end
